simulink model "two_parallel_full_model_simscape_ver_ii"  (R2023b)
settings: Solver=ode1be  StartTime=0.0  StopTime=simlength  FixedStep=ts_sim  MaxStep=ts_sim
undefined symbols (not defined in the file): fclock, fPWM_INV, fPWM_ZVS, gate_nominal_voltage, I_FS, Iout_dc_nom, ki_i_inv, ki_i_zvs, ki_v_inv, ki_v_zvs, kp_i_inv, kp_i_zvs, kp_v_inv, kp_v_zvs, LFi_dc, LFu_ac, magnitude, n10, omega_grid, pll_i1, pll_p, q1kalman, q2kalman, RCFu_dc, Rkalman, RLFi_dc, RLFu_ac, tc, Tc, tPWM_ZVS, ts_afe, ts_inv, ts_zvs, ugrid_factor, Ugrid_phase_normalization_factor, un_eta_pu, un_xi_pu, up_xi_pu, v1_trafo, v2_trafo, V_FS, Vnom_ac_adc, Vout_dc_nom, w
libraries: fl_lib x142, nesl_utility x55, single_phase_transformer_lib x4
(part 3 of 5)

== system two_parallel_full_model_simscape_ver_ii/inverter_modA/single phase inverter/switch_3 ==
  Diode : fl_lib/Electrical/Electrical Elements/Diode  Vf=Vdon_diode V  Ron=Rdon_diode Ohm  Goff=1e-8 1/Ohm  i_specify=off  i_priority=None  i=0 A  i_nominal_specify=off  i_nominal_unit=A  i_nominal_value=1  v_specify=off  v_priority=None  v=0 V  v_nominal_specify=off  v_nominal_unit=V  v_nominal_value=1
  Switch : fl_lib/Electrical/Electrical Elements/Switch  R_closed=Ron Ohm  G_open=1e-8 1/Ohm  Threshold=7.5  i_specify=off  i_priority=None  i=0 A  i_nominal_specify=off  i_nominal_unit=A  i_nominal_value=1  v_specify=off  v_priority=None  v=0 V  v_nominal_specify=off  v_nominal_unit=V  v_nominal_value=1
  G : PMIOPort  Side=Left
  C : PMIOPort  Port=2  Side=Left
  E : PMIOPort  Port=3  Side=Right
  connections:
  Switch/RConn2 -- C/RConn1 -- Diode/RConn1
  Switch/RConn1 -- G/RConn1
  Switch/LConn1 -- E/RConn1 -- Diode/LConn1

== system two_parallel_full_model_simscape_ver_ii/inverter_modA/single phase inverter/switch_4 ==
  Diode : fl_lib/Electrical/Electrical Elements/Diode  Vf=Vdon_diode V  Ron=Rdon_diode Ohm  Goff=1e-8 1/Ohm  i_specify=off  i_priority=None  i=0 A  i_nominal_specify=off  i_nominal_unit=A  i_nominal_value=1  v_specify=off  v_priority=None  v=0 V  v_nominal_specify=off  v_nominal_unit=V  v_nominal_value=1
  Switch : fl_lib/Electrical/Electrical Elements/Switch  R_closed=Ron Ohm  G_open=1e-8 1/Ohm  Threshold=7.5  i_specify=off  i_priority=None  i=0 A  i_nominal_specify=off  i_nominal_unit=A  i_nominal_value=1  v_specify=off  v_priority=None  v=0 V  v_nominal_specify=off  v_nominal_unit=V  v_nominal_value=1
  G : PMIOPort  Side=Left
  C : PMIOPort  Port=2  Side=Left
  E : PMIOPort  Port=3  Side=Right
  connections:
  Diode/LConn1 -- E/RConn1 -- Switch/LConn1
  Switch/RConn1 -- G/RConn1
  Diode/RConn1 -- C/RConn1 -- Switch/RConn2

== system two_parallel_full_model_simscape_ver_ii/inverter_modA/single phase inverter control/acquisition_and_scaling_current ==
  in : Inport
  1/Ti5 : Gain  Gain=1/I_FS  SaturateOnIntegerOverflow=on  OutDataTypeStr=Inherit: Same as input  ParamDataTypeStr=Inherit: Same as input
  Unit Delay4 : UnitDelay  SampleTime=ts_inv  HasFrameUpgradeWarning=on
  Zero-Order Hold1 : ZeroOrderHold  SampleTime=ts_inv
  out : Outport
  wires:
  in/1 -> Zero-Order Hold1/1
  1/Ti5/1 -> Unit Delay4/1
  Zero-Order Hold1/1 -> 1/Ti5/1
  Unit Delay4/1 -> out/1

== system two_parallel_full_model_simscape_ver_ii/inverter_modA/single phase inverter control/acquisition_and_scaling_voltage ==
  in : Inport
  1/Ti1 : Gain  Gain=1/V_FS  SaturateOnIntegerOverflow=on  OutDataTypeStr=Inherit: Same as input  ParamDataTypeStr=Inherit: Same as input
  Unit Delay4 : UnitDelay  SampleTime=ts_inv  HasFrameUpgradeWarning=on
  Zero-Order Hold2 : ZeroOrderHold  SampleTime=ts_inv
  out : Outport
  wires:
  1/Ti1/1 -> Unit Delay4/1
  Zero-Order Hold2/1 -> 1/Ti1/1
  Unit Delay4/1 -> out/1
  in/1 -> Zero-Order Hold2/1

== system two_parallel_full_model_simscape_ver_ii/inverter_modA/single phase inverter control/alpha_beta_transformation_i ==
  in : Inport
  Constant1 : Constant  Value=w
  Constant3 : Constant  Value=q1kalman
  Constant4 : Constant  Value=q2kalman
  Constant5 : Constant  Value=Rkalman
  Constant6 : Constant  Value=ts_inv
  Gain : Gain  Gain=-1
  kalman_observer : MATLAB Function  TreatAsAtomicUnit=on  SystemSampleTime=ts_inv
  alpha : Outport
  beta : Outport  Port=2
  wires:
  Gain/1 -> beta/1
  kalman_observer/1(h1_hat) -> alpha/1
  kalman_observer/2(h2_hat) -> Gain/1
  Constant1/1 -> kalman_observer/2(w)
  in/1 -> kalman_observer/1(y)
  Constant6/1 -> kalman_observer/3(Ts)
  Constant5/1 -> kalman_observer/6(r)
  Constant3/1 -> kalman_observer/4(q1)
  Constant4/1 -> kalman_observer/5(q2)

== system two_parallel_full_model_simscape_ver_ii/inverter_modA/single phase inverter control/alpha_beta_transformation_u ==
  in : Inport
  Constant1 : Constant  Value=w
  Constant3 : Constant  Value=q1kalman
  Constant4 : Constant  Value=q2kalman
  Constant5 : Constant  Value=Rkalman
  Constant6 : Constant  Value=ts_inv
  Gain : Gain  Gain=-1
  kalman_observer : MATLAB Function  TreatAsAtomicUnit=on  SystemSampleTime=ts_inv
  alpha : Outport
  beta : Outport  Port=2
  wires:
  Constant4/1 -> kalman_observer/5(q2)
  Constant3/1 -> kalman_observer/4(q1)
  Constant5/1 -> kalman_observer/6(r)
  Constant6/1 -> kalman_observer/3(Ts)
  in/1 -> kalman_observer/1(y)
  Constant1/1 -> kalman_observer/2(w)
  kalman_observer/2(h2_hat) -> Gain/1
  kalman_observer/1(h1_hat) -> alpha/1
  Gain/1 -> beta/1

== system two_parallel_full_model_simscape_ver_ii/inverter_modA/single phase inverter control/alphabeta2dq ==
  note: va=V cos(wt)
      | vb=V cos(wt-2pi/3)
      | vc=V cos(wt+2pi/3)
  alpha : Inport
  beta : Inport  Port=2
  wt : Inport  Port=3
  Product{,1..3} (4 alike) : Product  RndMeth=Zero
  Sum : Sum
  Sum1 : Sum  Inputs=-+
  To Workspace1 : ToWorkspace  VariableName=id_pu_modA_sim  SampleTime=ts_inv
      settings: MaxDataPoints=Ns_inv
  To Workspace2 : ToWorkspace  VariableName=iq_pu_modA_sim  SampleTime=ts_inv
      settings: MaxDataPoints=Ns_inv
  Trigonometric Function : Trigonometry  Operator=cos
  Trigonometric Function1 : Trigonometry
  "d " : Outport  VectorParamsAs1DForOutWhenUnconnected=off
  "q " : Outport  Port=2  VectorParamsAs1DForOutWhenUnconnected=off
  wires:
  wt/1 -> Trigonometric Function1/1, Trigonometric Function/1
  Trigonometric Function/1 -> [cos]
  Trigonometric Function1/1 -> [sin]
  [cos] -> Product/1
  alpha/1 -> Product/2, Product2/2
  Product/1 -> Sum/1
  Product1/1 -> Sum/2
  [sin] -> Product1/1
  beta/1 -> Product1/2, Product3/2
  Sum/1 -> To Workspace1/1, "d "/1
  [sin] -> Product2/1
  Product2/1 -> Sum1/1
  Product3/1 -> Sum1/2
  [cos] -> Product3/1
  Sum1/1 -> To Workspace2/1, "q "/1

== system two_parallel_full_model_simscape_ver_ii/inverter_modA/single phase inverter control/dq2alphabeta ==
  d : Inport
  q : Inport  Port=2
  wt : Inport  Port=3
  Product{,1..3} (4 alike) : Product  RndMeth=Zero
  Sum : Sum  Inputs=+-
  Sum1 : Sum
  Trigonometric Function : Trigonometry  Operator=cos
  Trigonometric Function1 : Trigonometry
  alpha : Outport  VectorParamsAs1DForOutWhenUnconnected=off
  wires:
  [cos] -> Product3/1
  Product3/1 -> Sum1/2
  Product2/1 -> Sum1/1
  [sin] -> Product2/1
  Sum/1 -> alpha/1
  q/1 -> Product3/2, Product1/2
  [sin] -> Product1/1
  Product1/1 -> Sum/2
  Product/1 -> Sum/1
  d/1 -> Product2/2, Product/2
  [cos] -> Product/1
  Trigonometric Function1/1 -> [sin]
  Trigonometric Function/1 -> [cos]
  wt/1 -> Trigonometric Function/1, Trigonometric Function1/1

== system two_parallel_full_model_simscape_ver_ii/inverter_modA/single phase inverter control/pi_d ==
  id_tilde : Inport
  1/Ti : Gain  Gain=kp_i_inv  SaturateOnIntegerOverflow=on  OutDataTypeStr=Inherit: Same as input  ParamDataTypeStr=Inherit: Same as input
  Sum1 : Sum  Inputs=+++  SaturateOnIntegerOverflow=on
  Sum3 : Sum  Inputs=-+  SaturateOnIntegerOverflow=on
  To Workspace3 : ToWorkspace  VariableName=id_ctrl_out_modA_sim  SampleTime=ts_inv
      settings: MaxDataPoints=Ns_inv
  Unit Delay4 : UnitDelay  SampleTime=ts_inv  HasFrameUpgradeWarning=on
  kp2 : Gain  Gain=ki_i_inv*ts_inv  SaturateOnIntegerOverflow=on  OutDataTypeStr=Inherit: Same as input  ParamDataTypeStr=Inherit: Same as input
  ud_out_lim : Saturate  UpperLimit=1  LowerLimit=-1
  "ud_out_lim " : Saturate  UpperLimit=1  LowerLimit=-1
  Vd_out : Outport  VectorParamsAs1DForOutWhenUnconnected=off
  wires:
  id_tilde/1 -> kp2/1, 1/Ti/1
  Sum1/1 -> ud_out_lim/1
  kp2/1 -> Sum1/2
  1/Ti/1 -> Sum1/1, Sum3/1
  Unit Delay4/1 -> Sum1/3
  Sum3/1 -> Unit Delay4/1
  ud_out_lim/1 -> Sum3/2, "ud_out_lim "/1
  "ud_out_lim "/1 -> To Workspace3/1, Vd_out/1

== system two_parallel_full_model_simscape_ver_ii/inverter_modA/single phase inverter control/pi_q ==
  iq_tilde : Inport
  1/Ti : Gain  Gain=kp_i_inv  SaturateOnIntegerOverflow=on  OutDataTypeStr=Inherit: Same as input  ParamDataTypeStr=Inherit: Same as input
  Sum1 : Sum  Inputs=+++  SaturateOnIntegerOverflow=on
  Sum3 : Sum  Inputs=-+  SaturateOnIntegerOverflow=on
  To Workspace3 : ToWorkspace  VariableName=iq_ctrl_out_modA_sim  SampleTime=ts_inv
      settings: MaxDataPoints=Ns_inv
  Unit Delay4 : UnitDelay  SampleTime=ts_inv  HasFrameUpgradeWarning=on
  kp2 : Gain  Gain=ki_i_inv*ts_inv  SaturateOnIntegerOverflow=on  OutDataTypeStr=Inherit: Same as input  ParamDataTypeStr=Inherit: Same as input
  ud_out_lim : Saturate  UpperLimit=1  LowerLimit=-1
  "uq_out_lim " : Saturate  UpperLimit=1  LowerLimit=-1
  Vd_out : Outport  VectorParamsAs1DForOutWhenUnconnected=off
  wires:
  "uq_out_lim "/1 -> Vd_out/1, To Workspace3/1
  ud_out_lim/1 -> "uq_out_lim "/1, Sum3/2
  Sum3/1 -> Unit Delay4/1
  Unit Delay4/1 -> Sum1/3
  1/Ti/1 -> Sum3/1, Sum1/1
  kp2/1 -> Sum1/2
  Sum1/1 -> ud_out_lim/1
  iq_tilde/1 -> 1/Ti/1, kp2/1

== system two_parallel_full_model_simscape_ver_ii/inverter_modA/single phase inverter control/pi_v ==
  e : Inport
  1/Ti : Gain  Gain=kp_v_inv  SaturateOnIntegerOverflow=on  OutDataTypeStr=Inherit: Same as input  ParamDataTypeStr=Inherit: Same as input
  Sum1 : Sum  Inputs=+++  SaturateOnIntegerOverflow=on
  Sum3 : Sum  Inputs=-+  SaturateOnIntegerOverflow=on
  To Workspace3 : ToWorkspace  VariableName=v_ctrl_out_modA_sim  SampleTime=ts_inv
      settings: MaxDataPoints=Ns_inv
  Unit Delay4 : UnitDelay  SampleTime=ts_inv  HasFrameUpgradeWarning=on
  i_out_lim : Saturate  UpperLimit=0.869565217391304  LowerLimit=0
  kp2 : Gain  Gain=ki_v_inv*ts_inv  SaturateOnIntegerOverflow=on  OutDataTypeStr=Inherit: Same as input  ParamDataTypeStr=Inherit: Same as input
  i_ref_internal : Outport  VectorParamsAs1DForOutWhenUnconnected=off
  wires:
  i_out_lim/1 -> i_ref_internal/1, To Workspace3/1, Sum3/2
  Sum3/1 -> Unit Delay4/1
  Unit Delay4/1 -> Sum1/3
  1/Ti/1 -> Sum3/1, Sum1/1
  kp2/1 -> Sum1/2
  Sum1/1 -> i_out_lim/1
  e/1 -> kp2/1, 1/Ti/1

== system two_parallel_full_model_simscape_ver_ii/inverter_modA/single phase inverter control/pwm ==
  vout : Inport
  Constant : Constant  Value=0
  Constant1 : Constant
  Constant2 : Constant
  Constant3 : Constant
  Gain1 : Gain  Gain=1/2
  Gain2 : Gain
  Gain3 : Gain  Gain=1/2
  Gain4 : Gain  Gain=-1
  PWM generator 1 : Subsystem  mask{f=fPWM_INV, m_up=1, m_low=0, dead_time=0, pos_cmd_gate=15, neg_cmd_gate=-10, polarity=-1}
      mask prompts: f "Frequency (Hz)"; m_up "Max Input Modulation Value"; m_low "Min Input Modulation Value"; dead_time "Dead Time (s)"; pos_cmd_gate "Positive Gate Voltage (V)"; neg_cmd_gate "Negative Gate Voltage (V)"; polarity "Polarity (pu)"
  PWM generator 2 : Subsystem  mask{f=fPWM_INV, m_up=1, m_low=0, dead_time=0, pos_cmd_gate=15, neg_cmd_gate=-10, polarity=-1}
      mask prompts: f "Frequency (Hz)"; m_up "Max Input Modulation Value"; m_low "Min Input Modulation Value"; dead_time "Dead Time (s)"; pos_cmd_gate "Positive Gate Voltage (V)"; neg_cmd_gate "Negative Gate Voltage (V)"; polarity "Polarity (pu)"
  Sum : Sum  Inputs=|++
  Sum1 : Sum  Inputs=|++
  m1_top : Outport
  m1_bottom : Outport  Port=2
  m2_top : Outport  Port=3
  m2_bottom : Outport  Port=4
  wires:
  PWM generator 1/1(m1) -> m1_top/1  "gate_cmd_Q1"
  PWM generator 1/2(m2) -> m1_bottom/1  "gate_cmd_Q2"
  PWM generator 2/2(m2) -> m2_bottom/1  "gate_cmd_Q2"
  PWM generator 2/1(m1) -> m2_top/1  "gate_cmd_Q1"
  Constant/1 -> PWM generator 2/2(phase), PWM generator 1/2(phase)
  Constant1/1 -> PWM generator 2/3(polarity_input), PWM generator 1/3(polarity_input)
  Gain2/1 -> Sum/1
  Sum/1 -> Gain1/1
  Constant2/1 -> Sum/2
  Gain1/1 -> PWM generator 1/1(m_index)
  Constant3/1 -> Sum1/2
  Sum1/1 -> Gain3/1
  Gain4/1 -> Sum1/1
  Gain3/1 -> PWM generator 2/1(m_index)
  vout/1 -> Gain4/1, Gain2/1

== system two_parallel_full_model_simscape_ver_ii/inverter_modB/pll_stageA/abc2alphabeta ==
  Vgrid_a : Inport
  Vgrid_b : Inport  Port=2
  Vgrid_c : Inport  Port=3
  Gain1 : Gain  Gain=1/Vnom_ac_adc
  Gain2 : Gain  Gain=1/Vnom_ac_adc
  Gain3 : Gain  Gain=1/Vnom_ac_adc
  Sum : Sum  Inputs=--|
  Terminator : Terminator
  Zero-Order Hold : ZeroOrderHold  SampleTime=ts_inv
  Zero-Order Hold1 : ZeroOrderHold  SampleTime=ts_inv
  Zero-Order Hold2 : ZeroOrderHold  SampleTime=ts_inv
  abc2alphabeta : Subsystem
  Vgrid_alpha : Outport  VectorParamsAs1DForOutWhenUnconnected=off
  Vgrid_beta : Outport  Port=2  VectorParamsAs1DForOutWhenUnconnected=off
  wires:
  abc2alphabeta/1("alpha ") -> Vgrid_alpha/1
  Vgrid_a/1 -> Zero-Order Hold/1
  Zero-Order Hold/1 -> Gain1/1
  abc2alphabeta/2("beta ") -> Vgrid_beta/1
  Zero-Order Hold1/1 -> Gain2/1
  Zero-Order Hold2/1 -> Gain3/1
  Vgrid_b/1 -> Zero-Order Hold1/1
  Vgrid_c/1 -> Zero-Order Hold2/1
  Gain1/1 -> Sum/2, abc2alphabeta/1(a)
  Gain2/1 -> Sum/1, abc2alphabeta/2(b)
  Sum/1 -> abc2alphabeta/3(c)
  Gain3/1 -> Terminator/1

== system two_parallel_full_model_simscape_ver_ii/inverter_modB/pll_stageB/alphabeta2xieta ==
  alpha : Inport
  beta : Inport  Port=2
  wt : Inport  Port=3
  Product{,1..3} (4 alike) : Product  RndMeth=Zero
  Sum : Sum
  Sum1 : Sum  Inputs=-+
  Trigonometric Function : Trigonometry  Operator=cos
  Trigonometric Function1 : Trigonometry
  xi : Outport  VectorParamsAs1DForOutWhenUnconnected=off
  eta : Outport  Port=2  VectorParamsAs1DForOutWhenUnconnected=off
  wires:
  Trigonometric Function/1 -> [cos]
  Trigonometric Function1/1 -> [sin]
  wt/1 -> Trigonometric Function1/1, Trigonometric Function/1
  Sum1/1 -> eta/1
  Sum/1 -> xi/1
  [cos] -> Product3/1
  Product3/1 -> Sum1/2
  Product2/1 -> Sum1/1
  [sin] -> Product2/1
  beta/1 -> Product3/2, Product1/2
  [sin] -> Product1/1
  Product1/1 -> Sum/2
  Product/1 -> Sum/1
  alpha/1 -> Product2/2, Product/2
  [cos] -> Product/1

== system two_parallel_full_model_simscape_ver_ii/inverter_modB/pll_stageB/pll_2 ==
  eta : Inport
  -2<x<2 : Saturate  UpperLimit=2  LowerLimit=-2
  Constant3 : Constant  Value=0
  Constant4 : Constant  Value=omega_grid
  Constant7 : Constant
  Product1 : Product  RndMeth=Zero
  Product2 : Product  RndMeth=Zero
  Sum1 : Sum  Inputs=|-+
  Sum3 : Sum  SaturateOnIntegerOverflow=on
  Sum4 : Sum  SaturateOnIntegerOverflow=on
  Sum5 : Sum  Inputs=+++
  Unit Delay1 : UnitDelay  SampleTime=ts_inv  HasFrameUpgradeWarning=on
  Unit Delay4 : UnitDelay  SampleTime=ts_inv  HasFrameUpgradeWarning=on
  bounder1 : MATLAB Function  TreatAsAtomicUnit=on  SystemSampleTime=ts_inv
  kp : Gain  Gain=pll_i1*ts_inv  SaturateOnIntegerOverflow=on  OutDataTypeStr=Inherit: Same as input  ParamDataTypeStr=Inherit: Same as input
  kp1 : Gain  Gain=pll_p  SaturateOnIntegerOverflow=on  OutDataTypeStr=Inherit: Same as input  ParamDataTypeStr=Inherit: Same as input
  kp2 : Gain  Gain=ts_inv  SaturateOnIntegerOverflow=on  OutDataTypeStr=Inherit: Same as input  ParamDataTypeStr=Inherit: Same as input
  kp3 : Gain  Gain=-1  SaturateOnIntegerOverflow=on  OutDataTypeStr=Inherit: Same as input  ParamDataTypeStr=Inherit: Same as input
  theta_est : Outport  VectorParamsAs1DForOutWhenUnconnected=off
  wires:
  Constant7/1 -> Sum5/3
  Constant3/1 -> Sum1/2
  [Vgrid_unorm_modB] -> Product1/2
  Product2/1 -> kp2/1
  kp/1 -> Sum3/1
  kp1/1 -> Sum5/1
  Product1/1 -> Sum1/1
  Sum1/1 -> kp3/1
  -2<x<2/1 -> Sum5/2, Unit Delay4/1  "i1"
  Unit Delay4/1 -> Sum3/2
  Sum3/1 -> -2<x<2/1
  kp2/1 -> Sum4/1
  Sum5/1 -> Product2/1
  Constant4/1 -> Product2/2
  Unit Delay1/1 -> Sum4/2, theta_est/1
  eta/1 -> Product1/1
  kp3/1 -> kp/1, kp1/1
  Sum4/1 -> bounder1/1(u)
  bounder1/1(y) -> Unit Delay1/1  "grid_emu_phase"

== system two_parallel_full_model_simscape_ver_ii/inverter_modB/single phase inverter/switch_1 ==
  Diode : fl_lib/Electrical/Electrical Elements/Diode  Vf=Vdon_diode V  Ron=Rdon_diode Ohm  Goff=1e-8 1/Ohm  i_specify=off  i_priority=None  i=0 A  i_nominal_specify=off  i_nominal_unit=A  i_nominal_value=1  v_specify=off  v_priority=None  v=0 V  v_nominal_specify=off  v_nominal_unit=V  v_nominal_value=1
  Switch : fl_lib/Electrical/Electrical Elements/Switch  R_closed=Ron Ohm  G_open=1e-8 1/Ohm  Threshold=7.5  i_specify=off  i_priority=None  i=0 A  i_nominal_specify=off  i_nominal_unit=A  i_nominal_value=1  v_specify=off  v_priority=None  v=0 V  v_nominal_specify=off  v_nominal_unit=V  v_nominal_value=1
  G : PMIOPort  Side=Left
  C : PMIOPort  Port=2  Side=Left
  E : PMIOPort  Port=3  Side=Right
  connections:
  Diode/LConn1 -- E/RConn1 -- Switch/LConn1
  Switch/RConn1 -- G/RConn1
  Diode/RConn1 -- C/RConn1 -- Switch/RConn2

== system two_parallel_full_model_simscape_ver_ii/inverter_modB/single phase inverter/switch_2 ==
  Diode : fl_lib/Electrical/Electrical Elements/Diode  Vf=Vdon_diode V  Ron=Rdon_diode Ohm  Goff=1e-8 1/Ohm  i_specify=off  i_priority=None  i=0 A  i_nominal_specify=off  i_nominal_unit=A  i_nominal_value=1  v_specify=off  v_priority=None  v=0 V  v_nominal_specify=off  v_nominal_unit=V  v_nominal_value=1
  Switch : fl_lib/Electrical/Electrical Elements/Switch  R_closed=Ron Ohm  G_open=1e-8 1/Ohm  Threshold=7.5  i_specify=off  i_priority=None  i=0 A  i_nominal_specify=off  i_nominal_unit=A  i_nominal_value=1  v_specify=off  v_priority=None  v=0 V  v_nominal_specify=off  v_nominal_unit=V  v_nominal_value=1
  G : PMIOPort  Side=Left
  C : PMIOPort  Port=2  Side=Left
  E : PMIOPort  Port=3  Side=Right
  connections:
  Switch/RConn2 -- C/RConn1 -- Diode/RConn1
  Switch/RConn1 -- G/RConn1
  Switch/LConn1 -- E/RConn1 -- Diode/LConn1

== system two_parallel_full_model_simscape_ver_ii/inverter_modB/single phase inverter/switch_3 ==
  Diode : fl_lib/Electrical/Electrical Elements/Diode  Vf=Vdon_diode V  Ron=Rdon_diode Ohm  Goff=1e-8 1/Ohm  i_specify=off  i_priority=None  i=0 A  i_nominal_specify=off  i_nominal_unit=A  i_nominal_value=1  v_specify=off  v_priority=None  v=0 V  v_nominal_specify=off  v_nominal_unit=V  v_nominal_value=1
  Switch : fl_lib/Electrical/Electrical Elements/Switch  R_closed=Ron Ohm  G_open=1e-8 1/Ohm  Threshold=7.5  i_specify=off  i_priority=None  i=0 A  i_nominal_specify=off  i_nominal_unit=A  i_nominal_value=1  v_specify=off  v_priority=None  v=0 V  v_nominal_specify=off  v_nominal_unit=V  v_nominal_value=1
  G : PMIOPort  Side=Left
  C : PMIOPort  Port=2  Side=Left
  E : PMIOPort  Port=3  Side=Right
  connections:
  Diode/LConn1 -- E/RConn1 -- Switch/LConn1
  Switch/RConn1 -- G/RConn1
  Diode/RConn1 -- C/RConn1 -- Switch/RConn2

== system two_parallel_full_model_simscape_ver_ii/inverter_modB/single phase inverter/switch_4 ==
  Diode : fl_lib/Electrical/Electrical Elements/Diode  Vf=Vdon_diode V  Ron=Rdon_diode Ohm  Goff=1e-8 1/Ohm  i_specify=off  i_priority=None  i=0 A  i_nominal_specify=off  i_nominal_unit=A  i_nominal_value=1  v_specify=off  v_priority=None  v=0 V  v_nominal_specify=off  v_nominal_unit=V  v_nominal_value=1
  Switch : fl_lib/Electrical/Electrical Elements/Switch  R_closed=Ron Ohm  G_open=1e-8 1/Ohm  Threshold=7.5  i_specify=off  i_priority=None  i=0 A  i_nominal_specify=off  i_nominal_unit=A  i_nominal_value=1  v_specify=off  v_priority=None  v=0 V  v_nominal_specify=off  v_nominal_unit=V  v_nominal_value=1
  G : PMIOPort  Side=Left
  C : PMIOPort  Port=2  Side=Left
  E : PMIOPort  Port=3  Side=Right
  connections:
  Switch/RConn2 -- C/RConn1 -- Diode/RConn1
  Switch/RConn1 -- G/RConn1
  Switch/LConn1 -- E/RConn1 -- Diode/LConn1

== system two_parallel_full_model_simscape_ver_ii/inverter_modB/single phase inverter control/acquisition_and_scaling_current ==
  in : Inport
  1/Ti5 : Gain  Gain=1/I_FS  SaturateOnIntegerOverflow=on  OutDataTypeStr=Inherit: Same as input  ParamDataTypeStr=Inherit: Same as input
  Unit Delay4 : UnitDelay  SampleTime=ts_inv  HasFrameUpgradeWarning=on
  Zero-Order Hold1 : ZeroOrderHold  SampleTime=ts_inv
  out : Outport
  wires:
  Unit Delay4/1 -> out/1
  Zero-Order Hold1/1 -> 1/Ti5/1
  1/Ti5/1 -> Unit Delay4/1
  in/1 -> Zero-Order Hold1/1

== system two_parallel_full_model_simscape_ver_ii/inverter_modB/single phase inverter control/alpha_beta_transformation_i ==
  in : Inport
  Constant1 : Constant  Value=w
  Constant3 : Constant  Value=q1kalman
  Constant4 : Constant  Value=q2kalman
  Constant5 : Constant  Value=Rkalman
  Constant6 : Constant  Value=ts_inv
  Gain : Gain  Gain=-1
  kalman_observer : MATLAB Function  TreatAsAtomicUnit=on  SystemSampleTime=ts_inv
  alpha : Outport
  beta : Outport  Port=2
  wires:
  Gain/1 -> beta/1
  kalman_observer/1(h1_hat) -> alpha/1
  kalman_observer/2(h2_hat) -> Gain/1
  Constant1/1 -> kalman_observer/2(w)
  in/1 -> kalman_observer/1(y)
  Constant6/1 -> kalman_observer/3(Ts)
  Constant5/1 -> kalman_observer/6(r)
  Constant3/1 -> kalman_observer/4(q1)
  Constant4/1 -> kalman_observer/5(q2)

== system two_parallel_full_model_simscape_ver_ii/inverter_modB/single phase inverter control/alphabeta2dq ==
  note: va=V cos(wt)
      | vb=V cos(wt-2pi/3)
      | vc=V cos(wt+2pi/3)
  alpha : Inport
  beta : Inport  Port=2
  wt : Inport  Port=3
  Product{,1..3} (4 alike) : Product  RndMeth=Zero
  Sum : Sum
  Sum1 : Sum  Inputs=-+
  To Workspace1 : ToWorkspace  VariableName=id_pu_modB_sim  SampleTime=ts_inv
      settings: MaxDataPoints=Ns_inv
  To Workspace2 : ToWorkspace  VariableName=iq_pu_modB_sim  SampleTime=ts_inv
      settings: MaxDataPoints=Ns_inv
  Trigonometric Function : Trigonometry  Operator=cos
  Trigonometric Function1 : Trigonometry
  "d " : Outport  VectorParamsAs1DForOutWhenUnconnected=off
  "q " : Outport  Port=2  VectorParamsAs1DForOutWhenUnconnected=off
  wires:
  Sum1/1 -> "q "/1, To Workspace2/1
  [cos] -> Product3/1
  Product3/1 -> Sum1/2
  Product2/1 -> Sum1/1
  [sin] -> Product2/1
  Sum/1 -> "d "/1, To Workspace1/1
  beta/1 -> Product3/2, Product1/2
  [sin] -> Product1/1
  Product1/1 -> Sum/2
  Product/1 -> Sum/1
  alpha/1 -> Product2/2, Product/2
  [cos] -> Product/1
  Trigonometric Function1/1 -> [sin]
  Trigonometric Function/1 -> [cos]
  wt/1 -> Trigonometric Function/1, Trigonometric Function1/1

== system two_parallel_full_model_simscape_ver_ii/inverter_modB/single phase inverter control/dq2alphabeta ==
  d : Inport
  q : Inport  Port=2
  wt : Inport  Port=3
  Product{,1..3} (4 alike) : Product  RndMeth=Zero
  Sum : Sum  Inputs=+-
  Sum1 : Sum
  Trigonometric Function : Trigonometry  Operator=cos
  Trigonometric Function1 : Trigonometry
  alpha : Outport  VectorParamsAs1DForOutWhenUnconnected=off
  wires:
  wt/1 -> Trigonometric Function1/1, Trigonometric Function/1
  Trigonometric Function/1 -> [cos]
  Trigonometric Function1/1 -> [sin]
  [cos] -> Product/1
  d/1 -> Product/2, Product2/2
  Product/1 -> Sum/1
  Product1/1 -> Sum/2
  [sin] -> Product1/1
  q/1 -> Product1/2, Product3/2
  Sum/1 -> alpha/1
  [sin] -> Product2/1
  Product2/1 -> Sum1/1
  Product3/1 -> Sum1/2
  [cos] -> Product3/1

== system two_parallel_full_model_simscape_ver_ii/inverter_modB/single phase inverter control/pi_d ==
  id_tilde : Inport
  1/Ti : Gain  Gain=kp_i_inv  SaturateOnIntegerOverflow=on  OutDataTypeStr=Inherit: Same as input  ParamDataTypeStr=Inherit: Same as input
  Sum1 : Sum  Inputs=+++  SaturateOnIntegerOverflow=on
  Sum3 : Sum  Inputs=-+  SaturateOnIntegerOverflow=on
  To Workspace3 : ToWorkspace  VariableName=id_ctrl_out_modB_sim  SampleTime=ts_inv
      settings: MaxDataPoints=Ns_inv
  Unit Delay4 : UnitDelay  SampleTime=ts_inv  HasFrameUpgradeWarning=on
  kp2 : Gain  Gain=ki_i_inv*ts_inv  SaturateOnIntegerOverflow=on  OutDataTypeStr=Inherit: Same as input  ParamDataTypeStr=Inherit: Same as input
  ud_out_lim : Saturate  UpperLimit=1  LowerLimit=-1
  "ud_out_lim " : Saturate  UpperLimit=1  LowerLimit=-1
  Vd_out : Outport  VectorParamsAs1DForOutWhenUnconnected=off
  wires:
  "ud_out_lim "/1 -> Vd_out/1, To Workspace3/1
  ud_out_lim/1 -> "ud_out_lim "/1, Sum3/2
  Sum3/1 -> Unit Delay4/1
  Unit Delay4/1 -> Sum1/3
  1/Ti/1 -> Sum3/1, Sum1/1
  kp2/1 -> Sum1/2
  Sum1/1 -> ud_out_lim/1
  id_tilde/1 -> 1/Ti/1, kp2/1

== system two_parallel_full_model_simscape_ver_ii/inverter_modB/single phase inverter control/pi_q ==
  iq_tilde : Inport
  1/Ti : Gain  Gain=kp_i_inv  SaturateOnIntegerOverflow=on  OutDataTypeStr=Inherit: Same as input  ParamDataTypeStr=Inherit: Same as input
  Sum1 : Sum  Inputs=+++  SaturateOnIntegerOverflow=on
  Sum3 : Sum  Inputs=-+  SaturateOnIntegerOverflow=on
  To Workspace3 : ToWorkspace  VariableName=iq_ctrl_out_modB_sim  SampleTime=ts_inv
      settings: MaxDataPoints=Ns_inv
  Unit Delay4 : UnitDelay  SampleTime=ts_inv  HasFrameUpgradeWarning=on
  kp2 : Gain  Gain=ki_i_inv*ts_inv  SaturateOnIntegerOverflow=on  OutDataTypeStr=Inherit: Same as input  ParamDataTypeStr=Inherit: Same as input
  ud_out_lim : Saturate  UpperLimit=1  LowerLimit=-1
  "uq_out_lim " : Saturate  UpperLimit=1  LowerLimit=-1
  Vd_out : Outport  VectorParamsAs1DForOutWhenUnconnected=off
  wires:
  Sum1/1 -> ud_out_lim/1
  kp2/1 -> Sum1/2
  1/Ti/1 -> Sum1/1, Sum3/1
  Unit Delay4/1 -> Sum1/3
  Sum3/1 -> Unit Delay4/1
  ud_out_lim/1 -> Sum3/2, "uq_out_lim "/1
  "uq_out_lim "/1 -> To Workspace3/1, Vd_out/1
  iq_tilde/1 -> kp2/1, 1/Ti/1

== system two_parallel_full_model_simscape_ver_ii/inverter_modB/single phase inverter control/pwm ==
  vout : Inport
  Constant : Constant  Value=-pi/24
  Constant1 : Constant
  Constant2 : Constant
  Constant3 : Constant
  Gain1 : Gain  Gain=1/2
  Gain2 : Gain
  Gain3 : Gain  Gain=1/2
  Gain4 : Gain  Gain=-1
  PWM generator 1 : Subsystem  mask{f=fPWM_INV, m_up=1, m_low=0, dead_time=0, pos_cmd_gate=15, neg_cmd_gate=-10, polarity=-1}
      mask prompts: f "Frequency (Hz)"; m_up "Max Input Modulation Value"; m_low "Min Input Modulation Value"; dead_time "Dead Time (s)"; pos_cmd_gate "Positive Gate Voltage (V)"; neg_cmd_gate "Negative Gate Voltage (V)"; polarity "Polarity (pu)"
  PWM generator 2 : Subsystem  mask{f=fPWM_INV, m_up=1, m_low=0, dead_time=0, pos_cmd_gate=15, neg_cmd_gate=-10, polarity=-1}
      mask prompts: f "Frequency (Hz)"; m_up "Max Input Modulation Value"; m_low "Min Input Modulation Value"; dead_time "Dead Time (s)"; pos_cmd_gate "Positive Gate Voltage (V)"; neg_cmd_gate "Negative Gate Voltage (V)"; polarity "Polarity (pu)"
  Sum : Sum  Inputs=|++
  Sum1 : Sum  Inputs=|++
  m1_top : Outport
  m1_bottom : Outport  Port=2
  m2_top : Outport  Port=3
  m2_bottom : Outport  Port=4
  wires:
  PWM generator 1/1(m1) -> m1_top/1  "gate_cmd_Q1"
  PWM generator 1/2(m2) -> m1_bottom/1  "gate_cmd_Q2"
  PWM generator 2/2(m2) -> m2_bottom/1  "gate_cmd_Q2"
  PWM generator 2/1(m1) -> m2_top/1  "gate_cmd_Q1"
  Constant/1 -> PWM generator 2/2(phase), PWM generator 1/2(phase)
  Constant1/1 -> PWM generator 2/3(polarity_input), PWM generator 1/3(polarity_input)
  Gain2/1 -> Sum/1
  Sum/1 -> Gain1/1
  Constant2/1 -> Sum/2
  Gain1/1 -> PWM generator 1/1(m_index)
  Constant3/1 -> Sum1/2
  Sum1/1 -> Gain3/1
  Gain4/1 -> Sum1/1
  Gain3/1 -> PWM generator 2/1(m_index)
  vout/1 -> Gain4/1, Gain2/1

== system two_parallel_full_model_simscape_ver_ii/zvs_modA/dc//dc with galvanic isolation/stage-1 ==
  gate_commands : Inport
  Current Sensor : fl_lib/Electrical/Electrical Sensors/Current Sensor
  PS-Simulink Converter1 : nesl_utility/PS-Simulink Converter  PhysicalDomain=network_engine_domain  SubClassName=ps_output  LeftPortType=input  RightPortType=output  PseudoPeriodic=off  Frequencies=[]  VectorFormat=1-D array  Unit=A  AffineConversion=on
  PS-Simulink Converter4 : nesl_utility/PS-Simulink Converter  PhysicalDomain=network_engine_domain  SubClassName=ps_output  LeftPortType=input  RightPortType=output  PseudoPeriodic=off  Frequencies=[]  VectorFormat=1-D array  Unit=V  AffineConversion=on
  Voltage Sensor : fl_lib/Electrical/Electrical Sensors/Voltage Sensor
  h-bridge : Subsystem
  uac_1(+) : PMIOPort  Side=Left
  uac_1(-) : PMIOPort  Port=2  Side=Left
  Udc(+) : PMIOPort  Port=3  Side=Right
  Udc(-) : PMIOPort  Port=4  Side=Right
  wires:
  gate_commands/1 -> h-bridge/1(gate_commands)
  connections:
  PS-Simulink Converter4/LConn1 -- Voltage Sensor/RConn1
  uac_1(+)/RConn1 -- h-bridge/LConn1
  uac_1(-)/RConn1 -- h-bridge/LConn2
  Voltage Sensor/RConn2 -- h-bridge/RConn2 -- Udc(-)/RConn1
  Current Sensor/LConn1 -- Udc(+)/RConn1
  Voltage Sensor/LConn1 -- h-bridge/RConn1 -- Current Sensor/RConn2
  PS-Simulink Converter1/LConn1 -- Current Sensor/RConn1

== system two_parallel_full_model_simscape_ver_ii/zvs_modA/dc//dc with galvanic isolation/stage-2 ==
  LFu1_dc{1..4} (4 alike) : fl_lib/Electrical/Electrical Elements/Inductor  l=LFu_dc H  r=RLFu_dc Ohm  g=1e-9 1/Ohm  i_specify=on  i_priority=High  i=0 A  i_nominal_specify=off  i_nominal_unit=A  i_nominal_value=1  v_specify=off  v_priority=None  v=0 V  v_nominal_specify=off  v_nominal_unit=V  v_nominal_value=1  i_L_specify=off  i_L_priority=High  i_L=0 A  i_L_nominal_specify=off  i_L_nominal_unit=A  i_L_nominal_value=1
  tr1 : single_phase_transformer_lib/single phase transformer  Lm=lm_trafo H  n1=1  n2=v2_trafo/v1_trafo  Rd1=0 Ohm  Rd2=rd2_trafo Ohm  Ld1=0 H  Ld2=ld2_trafo H  Rfe=rfe_trafo Ohm  phi_specify=off  phi_priority=None  phi=0 V*s  phi_nominal_specify=off  phi_nominal_unit=V*s  phi_nominal_value=1  i1_specify=off  i1_priority=None  i1=0 A  i1_nominal_specify=off  i1_nominal_unit=A  i1_nominal_value=1  i2_specify=off  i2_priority=None  i2=0 A  i2_nominal_specify=off  i2_nominal_unit=A  i2_nominal_value=1  ife_specify=off  ife_priority=None  ife=0 A  ife_nominal_specify=off  ife_nominal_unit=A  ife_nominal_value=1  u1_specify=off  u1_priority=None  u1=0 V  u1_nominal_specify=off  u1_nominal_unit=V  u1_nominal_value=1  u2_specify=off  u2_priority=None  u2=0 V  u2_nominal_specify=off  u2_nominal_unit=V  u2_nominal_value=1
      settings: InternalSimscapePortConfiguration="{\"Bottom\":[],\"Left\":[{\"id\":\"u1_p\",\"label\":\"u1(+)\",\"type\":\"foundation.electrical.electrical\"},{\"id\":\"u1_n\",\"label\":\"u1(-)\",\"type\":\"foundation.electrical.electrical\"}],\"Right\":[{\"id\":\"u2_p\",\"label\":\"u2(+)\",\"type\":\"foundation.electrical.electrical\"},{\"id\":\"u2_n\",\"label\":\"u2(-)\",\"type\":\"foundation.electrical.electrical\"}],\"Top\":[]}"
  tr2 : single_phase_transformer_lib/single phase transformer  Lm=lm_trafo H  n1=1  n2=v2_trafo/v1_trafo  Rd1=0 Ohm  Rd2=rd2_trafo Ohm  Ld1=0 H  Ld2=ld2_trafo H  Rfe=rfe_trafo Ohm  phi_specify=off  phi_priority=None  phi=0 V*s  phi_nominal_specify=off  phi_nominal_unit=V*s  phi_nominal_value=1  i1_specify=off  i1_priority=None  i1=0 A  i1_nominal_specify=off  i1_nominal_unit=A  i1_nominal_value=1  i2_specify=off  i2_priority=None  i2=0 A  i2_nominal_specify=off  i2_nominal_unit=A  i2_nominal_value=1  ife_specify=off  ife_priority=None  ife=0 A  ife_nominal_specify=off  ife_nominal_unit=A  ife_nominal_value=1  u1_specify=off  u1_priority=None  u1=0 V  u1_nominal_specify=off  u1_nominal_unit=V  u1_nominal_value=1  u2_specify=off  u2_priority=None  u2=0 V  u2_nominal_specify=off  u2_nominal_unit=V  u2_nominal_value=1
      settings: InternalSimscapePortConfiguration="{\"Bottom\":[],\"Left\":[{\"id\":\"u1_p\",\"label\":\"u1(+)\",\"type\":\"foundation.electrical.electrical\"},{\"id\":\"u1_n\",\"label\":\"u1(-)\",\"type\":\"foundation.electrical.electrical\"}],\"Right\":[{\"id\":\"u2_p\",\"label\":\"u2(+)\",\"type\":\"foundation.electrical.electrical\"},{\"id\":\"u2_n\",\"label\":\"u2(-)\",\"type\":\"foundation.electrical.electrical\"}],\"Top\":[]}"
  two-phase-rectifier_tr1 : Subsystem
  two-phase-rectifier_tr2 : Subsystem
  uac_1(+) : PMIOPort  Side=Left
  udc(+) : PMIOPort  Port=2  Side=Right
  uac_1(-) : PMIOPort  Port=3  Side=Left
  udc_(-) : PMIOPort  Port=4  Side=Right
  connections:
  uac_1(+)/RConn1 -- tr1/LConn1 -- tr2/LConn1
  uac_1(-)/RConn1 -- tr2/LConn2 -- tr1/LConn2
  tr1/RConn1 -- two-phase-rectifier_tr1/LConn1
  two-phase-rectifier_tr2/LConn1 -- tr2/RConn1
  two-phase-rectifier_tr2/LConn2 -- tr2/RConn2
  tr1/RConn2 -- two-phase-rectifier_tr1/LConn2
  LFu1_dc1/LConn1 -- two-phase-rectifier_tr1/RConn1
  two-phase-rectifier_tr1/RConn2 -- LFu1_dc2/RConn1
  two-phase-rectifier_tr2/RConn1 -- LFu1_dc3/LConn1
  LFu1_dc2/LConn1 -- LFu1_dc3/RConn1
  two-phase-rectifier_tr2/RConn2 -- LFu1_dc4/RConn1
  LFu1_dc4/LConn1 -- udc_(-)/RConn1
  LFu1_dc1/RConn1 -- udc(+)/RConn1

== system two_parallel_full_model_simscape_ver_ii/zvs_modA/grid_rectifier/three-phase-rectifier ==
  Diode{,1..5} (6 alike) : fl_lib/Electrical/Electrical Elements/Diode  Vf=Vdon_diode V  Ron=Rdon_diode Ohm  Goff=1e-8 1/Ohm  i_specify=off  i_priority=None  i=0 A  i_nominal_specify=off  i_nominal_unit=A  i_nominal_value=1  v_specify=off  v_priority=None  v=0 V  v_nominal_specify=off  v_nominal_unit=V  v_nominal_value=1
  udc(+) : PMIOPort  Side=Right
  ua : PMIOPort  Port=2  Side=Left
  ub : PMIOPort  Port=3  Side=Left
  uc : PMIOPort  Port=4  Side=Left
  udc(-) : PMIOPort  Port=5  Side=Right
  connections:
  Diode/LConn1 -- ua/RConn1 -- Diode3/RConn1
  Diode/RConn1 -- udc(+)/RConn1 -- Diode2/RConn1 -- Diode1/RConn1
  Diode3/LConn1 -- Diode4/LConn1 -- udc(-)/RConn1 -- Diode5/LConn1
  Diode1/LConn1 -- ub/RConn1 -- Diode4/RConn1
  Diode5/RConn1 -- Diode2/LConn1 -- uc/RConn1

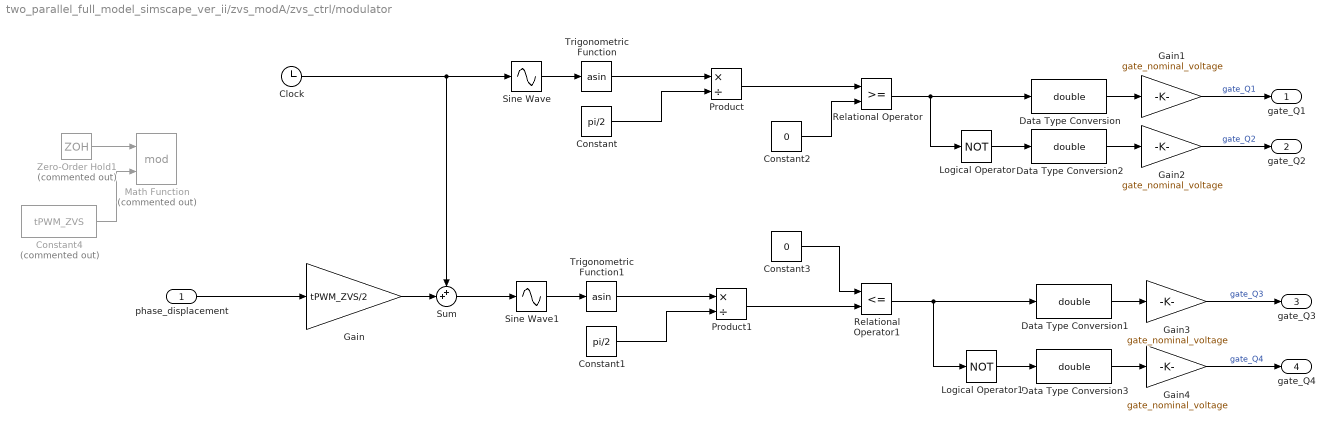
== system two_parallel_full_model_simscape_ver_ii/zvs_modA/zvs_ctrl/modulator ==
  phase_displacement : Inport
  Clock : Clock
  Constant : Constant  Value=pi/2
  Constant1 : Constant  Value=pi/2
  Constant2 : Constant  Value=0
  Constant3 : Constant  Value=0
  Constant4 : Constant  Commented=on  Value=tPWM_ZVS
  Data Type Conversion{,1..3} (4 alike) : DataTypeConversion  OutDataTypeStr=double  SaturateOnIntegerOverflow=off  RndMeth=Floor
  Gain : Gain  Gain=tPWM_ZVS/2  OutDataTypeStr=double
  Gain{1..4} (4 alike) : Gain  Gain=gate_nominal_voltage  OutDataTypeStr=double
  Logical Operator : Logic  Operator=NOT  AllPortsSameDT=off  OutDataTypeStr=boolean
  Logical Operator1 : Logic  Operator=NOT  AllPortsSameDT=off  OutDataTypeStr=boolean
  Math Function : Math  Commented=on  Operator=mod  SignedPower=on
  Product : Product  Inputs=*/
  Product1 : Product  Inputs=*/
  Relational Operator : RelationalOperator
  Relational Operator1 : RelationalOperator  Operator=<=
  Sine Wave : Sin  TimeSource=Use external signal  Frequency=2*pi*fPWM_ZVS
  Sine Wave1 : Sin  TimeSource=Use external signal  Frequency=2*pi*fPWM_ZVS
  Sum : Sum  Inputs=++|
  Trigonometric Function : Trigonometry  Operator=asin
  Trigonometric Function1 : Trigonometry  Operator=asin
  Zero-Order Hold1 : ZeroOrderHold  Commented=on  SampleTime=1/fclock
  gate_Q1 : Outport
  gate_Q2 : Outport  Port=2
  gate_Q3 : Outport  Port=3
  gate_Q4 : Outport  Port=4
  wires:
  Data Type Conversion/1 -> Gain1/1
  Data Type Conversion1/1 -> Gain3/1
  Sine Wave/1 -> Trigonometric Function/1
  Trigonometric Function/1 -> Product/1
  Constant/1 -> Product/2
  Product/1 -> Relational Operator/1
  Relational Operator/1 -> Logical Operator/1, Data Type Conversion/1
  Sine Wave1/1 -> Trigonometric Function1/1
  Trigonometric Function1/1 -> Product1/1
  Constant1/1 -> Product1/2
  Relational Operator1/1 -> Logical Operator1/1, Data Type Conversion1/1
  Product1/1 -> Relational Operator1/2
  Clock/1 -> Sum/1, Sine Wave/1
  Sum/1 -> Sine Wave1/1
  Constant2/1 -> Relational Operator/2
  Constant3/1 -> Relational Operator1/1
  Logical Operator/1 -> Data Type Conversion2/1
  Data Type Conversion2/1 -> Gain2/1
  Logical Operator1/1 -> Data Type Conversion3/1
  Data Type Conversion3/1 -> Gain4/1
  Gain/1 -> Sum/2
  phase_displacement/1 -> Gain/1
  Constant4/1 -> Math Function/2
  Zero-Order Hold1/1 -> Math Function/1
  Gain1/1 -> gate_Q1/1  "gate_Q1"
  Gain2/1 -> gate_Q2/1  "gate_Q2"
  Gain3/1 -> gate_Q3/1  "gate_Q3"
  Gain4/1 -> gate_Q4/1  "gate_Q4"

== system two_parallel_full_model_simscape_ver_ii/zvs_modA/zvs_ctrl/references ==
  voltage_reference : Subsystem
  vout_ref : Outport
  wires:
  voltage_reference/1(vout_ref) -> vout_ref/1

== system two_parallel_full_model_simscape_ver_ii/zvs_modA/zvs_ctrl/sampling_i_filter1 ==
  in : Inport
  1/Ti3 : Gain  Gain=1/I_FS  OutDataTypeStr=double  SaturateOnIntegerOverflow=on  ParamDataTypeStr=Inherit: Same as input
  Saturation : Saturate  UpperLimit=1  LowerLimit=0  OutDataTypeStr=double
  Zero-Order Hold2 : ZeroOrderHold  SampleTime=ts_zvs
  out_pu : Outport
  wires:
  in/1 -> 1/Ti3/1
  1/Ti3/1 -> Saturation/1
  Saturation/1 -> Zero-Order Hold2/1
  Zero-Order Hold2/1 -> out_pu/1

== system two_parallel_full_model_simscape_ver_ii/zvs_modA/zvs_ctrl/sampling_v_filter1 ==
  in : Inport
  1/Ti3 : Gain  Gain=1/V_FS  OutDataTypeStr=double  SaturateOnIntegerOverflow=on  ParamDataTypeStr=Inherit: Same as input
  Saturation : Saturate  UpperLimit=1  LowerLimit=0  OutDataTypeStr=double
  Zero-Order Hold2 : ZeroOrderHold  SampleTime=ts_zvs
  out_pu : Outport
  wires:
  Zero-Order Hold2/1 -> out_pu/1
  1/Ti3/1 -> Saturation/1
  in/1 -> 1/Ti3/1
  Saturation/1 -> Zero-Order Hold2/1

== system two_parallel_full_model_simscape_ver_ii/zvs_modA/zvs_ctrl/sampling_v_filter2 ==
  in : Inport
  1/Ti3 : Gain  Gain=1/V_FS  OutDataTypeStr=double  SaturateOnIntegerOverflow=on  ParamDataTypeStr=Inherit: Same as input
  Saturation : Saturate  UpperLimit=1  LowerLimit=0  OutDataTypeStr=double
  Zero-Order Hold2 : ZeroOrderHold  SampleTime=ts_zvs
  out_pu : Outport
  wires:
  in/1 -> 1/Ti3/1
  1/Ti3/1 -> Saturation/1
  Zero-Order Hold2/1 -> out_pu/1
  Saturation/1 -> Zero-Order Hold2/1

== system two_parallel_full_model_simscape_ver_ii/zvs_modA/zvs_ctrl/vi ctrl ==
  iout : Inport
  vout : Inport  Port=2
  vout_ref : Inport  Port=3
  Constant : Constant  Value=Iout_dc_nom
  Iout Ctrl : Subsystem
  Min : MinMax  Inputs=2
  To Workspace1 : ToWorkspace  VariableName=phase_ctrl_out_modA_sim  SampleTime=ts_zvs
      settings: MaxDataPoints=Ns_zvs
  To Workspace2 : ToWorkspace  VariableName=pid_ctrlv_out_modA_sim  SampleTime=ts_zvs
      settings: MaxDataPoints=Ns_zvs
  To Workspace3 : ToWorkspace  VariableName=pid_ctrli_out_modA_sim  SampleTime=ts_zvs
      settings: MaxDataPoints=Ns_zvs
  Unit Delay2 : UnitDelay  SampleTime=ts_zvs  HasFrameUpgradeWarning=on
  Vout Ctrl : Subsystem
  phase_displacement : Outport
  wires:
  Unit Delay2/1 -> phase_displacement/1, To Workspace1/1
  iout/1 -> Iout Ctrl/2(iout)
  vout_ref/1 -> Vout Ctrl/1(vout_ref)
  vout/1 -> Vout Ctrl/2(vout)
  Vout Ctrl/1(ctrlv_out) -> Min/1, To Workspace2/1
  Constant/1 -> Iout Ctrl/1(iout_ref)
  Iout Ctrl/1(ctrli_out) -> To Workspace3/1, Min/2
  Min/1 -> Unit Delay2/1

== system two_parallel_full_model_simscape_ver_ii/zvs_modB/dc//dc with galvanic isolation/stage-1 ==
  gate_commands : Inport
  Current Sensor : fl_lib/Electrical/Electrical Sensors/Current Sensor
  PS-Simulink Converter1 : nesl_utility/PS-Simulink Converter  PhysicalDomain=network_engine_domain  SubClassName=ps_output  LeftPortType=input  RightPortType=output  PseudoPeriodic=off  Frequencies=[]  VectorFormat=1-D array  Unit=A  AffineConversion=on
  PS-Simulink Converter4 : nesl_utility/PS-Simulink Converter  PhysicalDomain=network_engine_domain  SubClassName=ps_output  LeftPortType=input  RightPortType=output  PseudoPeriodic=off  Frequencies=[]  VectorFormat=1-D array  Unit=V  AffineConversion=on
  Voltage Sensor : fl_lib/Electrical/Electrical Sensors/Voltage Sensor
  h-bridge : Subsystem
  uac_1(+) : PMIOPort  Side=Left
  uac_1(-) : PMIOPort  Port=2  Side=Left
  Udc(+) : PMIOPort  Port=3  Side=Right
  Udc(-) : PMIOPort  Port=4  Side=Right
  wires:
  gate_commands/1 -> h-bridge/1(gate_commands)
  connections:
  PS-Simulink Converter1/LConn1 -- Current Sensor/RConn1
  Current Sensor/RConn2 -- h-bridge/RConn1 -- Voltage Sensor/LConn1
  Current Sensor/LConn1 -- Udc(+)/RConn1
  Udc(-)/RConn1 -- h-bridge/RConn2 -- Voltage Sensor/RConn2
  uac_1(-)/RConn1 -- h-bridge/LConn2
  uac_1(+)/RConn1 -- h-bridge/LConn1
  PS-Simulink Converter4/LConn1 -- Voltage Sensor/RConn1

== system two_parallel_full_model_simscape_ver_ii/zvs_modB/dc//dc with galvanic isolation/stage-2 ==
  LFu1_dc{1..4} (4 alike) : fl_lib/Electrical/Electrical Elements/Inductor  l=LFu_dc H  r=RLFu_dc Ohm  g=1e-9 1/Ohm  i_specify=on  i_priority=High  i=0 A  i_nominal_specify=off  i_nominal_unit=A  i_nominal_value=1  v_specify=off  v_priority=None  v=0 V  v_nominal_specify=off  v_nominal_unit=V  v_nominal_value=1  i_L_specify=off  i_L_priority=High  i_L=0 A  i_L_nominal_specify=off  i_L_nominal_unit=A  i_L_nominal_value=1
  tr1 : single_phase_transformer_lib/single phase transformer  Lm=lm_trafo H  n1=1  n2=v2_trafo/v1_trafo  Rd1=0 Ohm  Rd2=rd2_trafo Ohm  Ld1=0 H  Ld2=ld2_trafo H  Rfe=rfe_trafo Ohm  phi_specify=off  phi_priority=None  phi=0 V*s  phi_nominal_specify=off  phi_nominal_unit=V*s  phi_nominal_value=1  i1_specify=off  i1_priority=None  i1=0 A  i1_nominal_specify=off  i1_nominal_unit=A  i1_nominal_value=1  i2_specify=off  i2_priority=None  i2=0 A  i2_nominal_specify=off  i2_nominal_unit=A  i2_nominal_value=1  ife_specify=off  ife_priority=None  ife=0 A  ife_nominal_specify=off  ife_nominal_unit=A  ife_nominal_value=1  u1_specify=off  u1_priority=None  u1=0 V  u1_nominal_specify=off  u1_nominal_unit=V  u1_nominal_value=1  u2_specify=off  u2_priority=None  u2=0 V  u2_nominal_specify=off  u2_nominal_unit=V  u2_nominal_value=1
      settings: InternalSimscapePortConfiguration="{\"Bottom\":[],\"Left\":[{\"id\":\"u1_p\",\"label\":\"u1(+)\",\"type\":\"foundation.electrical.electrical\"},{\"id\":\"u1_n\",\"label\":\"u1(-)\",\"type\":\"foundation.electrical.electrical\"}],\"Right\":[{\"id\":\"u2_p\",\"label\":\"u2(+)\",\"type\":\"foundation.electrical.electrical\"},{\"id\":\"u2_n\",\"label\":\"u2(-)\",\"type\":\"foundation.electrical.electrical\"}],\"Top\":[]}"
  tr2 : single_phase_transformer_lib/single phase transformer  Lm=lm_trafo H  n1=1  n2=v2_trafo/v1_trafo  Rd1=0 Ohm  Rd2=rd2_trafo Ohm  Ld1=0 H  Ld2=ld2_trafo H  Rfe=rfe_trafo Ohm  phi_specify=off  phi_priority=None  phi=0 V*s  phi_nominal_specify=off  phi_nominal_unit=V*s  phi_nominal_value=1  i1_specify=off  i1_priority=None  i1=0 A  i1_nominal_specify=off  i1_nominal_unit=A  i1_nominal_value=1  i2_specify=off  i2_priority=None  i2=0 A  i2_nominal_specify=off  i2_nominal_unit=A  i2_nominal_value=1  ife_specify=off  ife_priority=None  ife=0 A  ife_nominal_specify=off  ife_nominal_unit=A  ife_nominal_value=1  u1_specify=off  u1_priority=None  u1=0 V  u1_nominal_specify=off  u1_nominal_unit=V  u1_nominal_value=1  u2_specify=off  u2_priority=None  u2=0 V  u2_nominal_specify=off  u2_nominal_unit=V  u2_nominal_value=1
      settings: InternalSimscapePortConfiguration="{\"Bottom\":[],\"Left\":[{\"id\":\"u1_p\",\"label\":\"u1(+)\",\"type\":\"foundation.electrical.electrical\"},{\"id\":\"u1_n\",\"label\":\"u1(-)\",\"type\":\"foundation.electrical.electrical\"}],\"Right\":[{\"id\":\"u2_p\",\"label\":\"u2(+)\",\"type\":\"foundation.electrical.electrical\"},{\"id\":\"u2_n\",\"label\":\"u2(-)\",\"type\":\"foundation.electrical.electrical\"}],\"Top\":[]}"
  two-phase-rectifier_tr1 : Subsystem
  two-phase-rectifier_tr2 : Subsystem
  uac_1(+) : PMIOPort  Side=Left
  udc(+) : PMIOPort  Port=2  Side=Right
  uac_1(-) : PMIOPort  Port=3  Side=Left
  udc_(-) : PMIOPort  Port=4  Side=Right
  connections:
  LFu1_dc1/RConn1 -- udc(+)/RConn1
  LFu1_dc4/LConn1 -- udc_(-)/RConn1
  two-phase-rectifier_tr2/RConn2 -- LFu1_dc4/RConn1
  LFu1_dc2/LConn1 -- LFu1_dc3/RConn1
  two-phase-rectifier_tr2/RConn1 -- LFu1_dc3/LConn1
  two-phase-rectifier_tr1/RConn2 -- LFu1_dc2/RConn1
  LFu1_dc1/LConn1 -- two-phase-rectifier_tr1/RConn1
  tr1/RConn2 -- two-phase-rectifier_tr1/LConn2
  two-phase-rectifier_tr2/LConn2 -- tr2/RConn2
  two-phase-rectifier_tr2/LConn1 -- tr2/RConn1
  tr1/RConn1 -- two-phase-rectifier_tr1/LConn1
  tr1/LConn2 -- tr2/LConn2 -- uac_1(-)/RConn1
  tr2/LConn1 -- tr1/LConn1 -- uac_1(+)/RConn1

== system two_parallel_full_model_simscape_ver_ii/zvs_modB/grid_rectifier/three-phase-rectifier ==
  Diode{,1..5} (6 alike) : fl_lib/Electrical/Electrical Elements/Diode  Vf=Vdon_diode V  Ron=Rdon_diode Ohm  Goff=1e-8 1/Ohm  i_specify=off  i_priority=None  i=0 A  i_nominal_specify=off  i_nominal_unit=A  i_nominal_value=1  v_specify=off  v_priority=None  v=0 V  v_nominal_specify=off  v_nominal_unit=V  v_nominal_value=1
  udc(+) : PMIOPort  Side=Right
  ua : PMIOPort  Port=2  Side=Left
  ub : PMIOPort  Port=3  Side=Left
  uc : PMIOPort  Port=4  Side=Left
  udc(-) : PMIOPort  Port=5  Side=Right
  connections:
  uc/RConn1 -- Diode2/LConn1 -- Diode5/RConn1
  Diode4/RConn1 -- ub/RConn1 -- Diode1/LConn1
  Diode5/LConn1 -- udc(-)/RConn1 -- Diode4/LConn1 -- Diode3/LConn1
  Diode1/RConn1 -- Diode2/RConn1 -- udc(+)/RConn1 -- Diode/RConn1
  Diode3/RConn1 -- ua/RConn1 -- Diode/LConn1

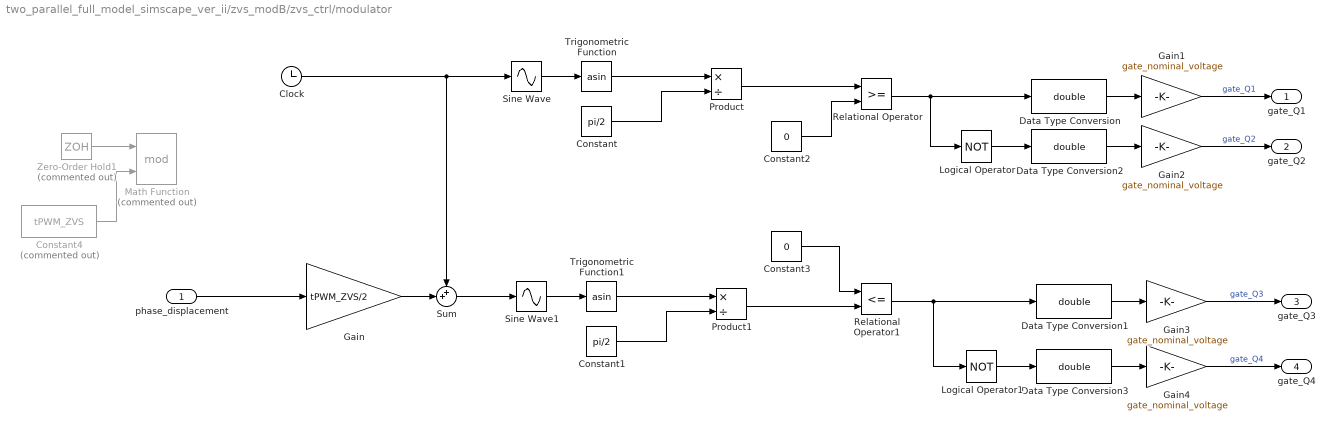
== system two_parallel_full_model_simscape_ver_ii/zvs_modB/zvs_ctrl/modulator ==
  phase_displacement : Inport
  Clock : Clock
  Constant : Constant  Value=pi/2
  Constant1 : Constant  Value=pi/2
  Constant2 : Constant  Value=0
  Constant3 : Constant  Value=0
  Constant4 : Constant  Commented=on  Value=tPWM_ZVS
  Data Type Conversion{,1..3} (4 alike) : DataTypeConversion  OutDataTypeStr=double  SaturateOnIntegerOverflow=off  RndMeth=Floor
  Gain : Gain  Gain=tPWM_ZVS/2  OutDataTypeStr=double
  Gain{1..4} (4 alike) : Gain  Gain=gate_nominal_voltage  OutDataTypeStr=double
  Logical Operator : Logic  Operator=NOT  AllPortsSameDT=off  OutDataTypeStr=boolean
  Logical Operator1 : Logic  Operator=NOT  AllPortsSameDT=off  OutDataTypeStr=boolean
  Math Function : Math  Commented=on  Operator=mod  SignedPower=on
  Product : Product  Inputs=*/
  Product1 : Product  Inputs=*/
  Relational Operator : RelationalOperator
  Relational Operator1 : RelationalOperator  Operator=<=
  Sine Wave : Sin  TimeSource=Use external signal  Frequency=2*pi*fPWM_ZVS
  Sine Wave1 : Sin  TimeSource=Use external signal  Frequency=2*pi*fPWM_ZVS
  Sum : Sum  Inputs=++|
  Trigonometric Function : Trigonometry  Operator=asin
  Trigonometric Function1 : Trigonometry  Operator=asin
  Zero-Order Hold1 : ZeroOrderHold  Commented=on  SampleTime=1/fclock
  gate_Q1 : Outport
  gate_Q2 : Outport  Port=2
  gate_Q3 : Outport  Port=3
  gate_Q4 : Outport  Port=4
  wires:
  Gain4/1 -> gate_Q4/1  "gate_Q4"
  Gain3/1 -> gate_Q3/1  "gate_Q3"
  Gain2/1 -> gate_Q2/1  "gate_Q2"
  Gain1/1 -> gate_Q1/1  "gate_Q1"
  Zero-Order Hold1/1 -> Math Function/1
  Constant4/1 -> Math Function/2
  phase_displacement/1 -> Gain/1
  Gain/1 -> Sum/2
  Data Type Conversion3/1 -> Gain4/1
  Logical Operator1/1 -> Data Type Conversion3/1
  Data Type Conversion2/1 -> Gain2/1
  Logical Operator/1 -> Data Type Conversion2/1
  Constant3/1 -> Relational Operator1/1
  Constant2/1 -> Relational Operator/2
  Sum/1 -> Sine Wave1/1
  Clock/1 -> Sine Wave/1, Sum/1
  Product1/1 -> Relational Operator1/2
  Relational Operator1/1 -> Data Type Conversion1/1, Logical Operator1/1
  Constant1/1 -> Product1/2
  Trigonometric Function1/1 -> Product1/1
  Sine Wave1/1 -> Trigonometric Function1/1
  Relational Operator/1 -> Data Type Conversion/1, Logical Operator/1
  Product/1 -> Relational Operator/1
  Constant/1 -> Product/2
  Trigonometric Function/1 -> Product/1
  Sine Wave/1 -> Trigonometric Function/1
  Data Type Conversion1/1 -> Gain3/1
  Data Type Conversion/1 -> Gain1/1

== system two_parallel_full_model_simscape_ver_ii/zvs_modB/zvs_ctrl/references ==
  voltage_reference : Subsystem
  vout_ref : Outport
  wires:
  voltage_reference/1(vout_ref) -> vout_ref/1

== system two_parallel_full_model_simscape_ver_ii/zvs_modB/zvs_ctrl/sampling_i_filter1 ==
  in : Inport
  1/Ti3 : Gain  Gain=1/I_FS  OutDataTypeStr=double  SaturateOnIntegerOverflow=on  ParamDataTypeStr=Inherit: Same as input
  Saturation : Saturate  UpperLimit=1  LowerLimit=0  OutDataTypeStr=double
  Zero-Order Hold2 : ZeroOrderHold  SampleTime=ts_zvs
  out_pu : Outport
  wires:
  Zero-Order Hold2/1 -> out_pu/1
  Saturation/1 -> Zero-Order Hold2/1
  1/Ti3/1 -> Saturation/1
  in/1 -> 1/Ti3/1

== system two_parallel_full_model_simscape_ver_ii/zvs_modB/zvs_ctrl/sampling_v_filter1 ==
  in : Inport
  1/Ti3 : Gain  Gain=1/V_FS  OutDataTypeStr=double  SaturateOnIntegerOverflow=on  ParamDataTypeStr=Inherit: Same as input
  Saturation : Saturate  UpperLimit=1  LowerLimit=0  OutDataTypeStr=double
  Zero-Order Hold2 : ZeroOrderHold  SampleTime=ts_zvs
  out_pu : Outport
  wires:
  Saturation/1 -> Zero-Order Hold2/1
  in/1 -> 1/Ti3/1
  1/Ti3/1 -> Saturation/1
  Zero-Order Hold2/1 -> out_pu/1

== system two_parallel_full_model_simscape_ver_ii/zvs_modB/zvs_ctrl/sampling_v_filter2 ==
  in : Inport
  1/Ti3 : Gain  Gain=1/V_FS  OutDataTypeStr=double  SaturateOnIntegerOverflow=on  ParamDataTypeStr=Inherit: Same as input
  Saturation : Saturate  UpperLimit=1  LowerLimit=0  OutDataTypeStr=double
  Zero-Order Hold2 : ZeroOrderHold  SampleTime=ts_zvs
  out_pu : Outport
  wires:
  Saturation/1 -> Zero-Order Hold2/1
  Zero-Order Hold2/1 -> out_pu/1
  1/Ti3/1 -> Saturation/1
  in/1 -> 1/Ti3/1
